simulink model "Disturbance"  (R2023b)
settings: Solver=VariableStepAuto  StartTime=0.0  StopTime=10.0  RelTol=1e-3
settings Model: Creator=hp  LastModifiedBy=hp

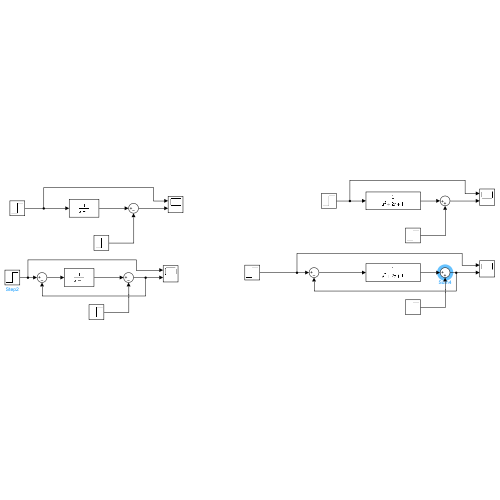
[thumbnail: Simulink's stored preview of the top-level diagram]
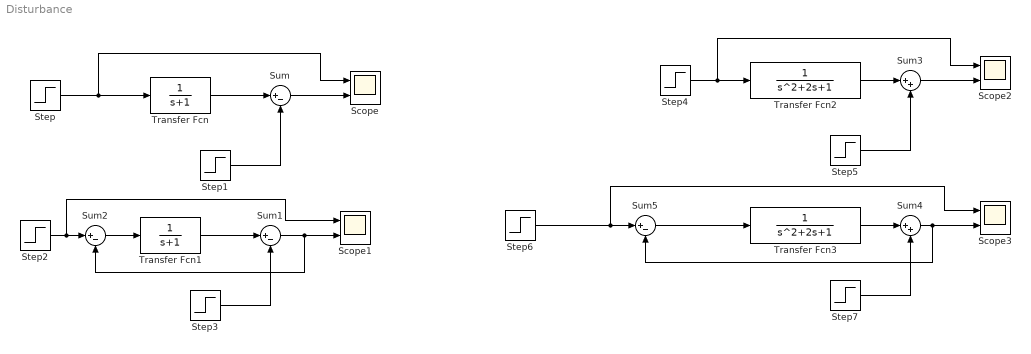
== system Disturbance ==
  Scope{,1..3} (4 alike) : Scope  NumInputPorts=2
  Step{,2,4,6} (4 alike) : Step  SampleTime=0
  Step1 : Step  Time=3  After=0.5  SampleTime=0
  Step3 : Step  Time=3  After=0.5  SampleTime=0
  Step5 : Step  Time=4  SampleTime=0.5
  Step7 : Step  Time=4  SampleTime=0.5
  Sum{,1..2,5} (4 alike) : Sum  Inputs=|+-
  Sum3 : Sum  Inputs=|++
  Sum4 : Sum  Inputs=|++
  Transfer Fcn : TransferFcn  Denominator=[1 1]
  Transfer Fcn1 : TransferFcn  Denominator=[1 1]
  Transfer Fcn2 : TransferFcn
  Transfer Fcn3 : TransferFcn
  wires:
  Transfer Fcn/1 -> Sum/1
  Sum/1 -> Scope/2
  Step1/1 -> Sum/2
  Step/1 -> Scope/1, Transfer Fcn/1
  Step3/1 -> Sum1/2
  Transfer Fcn1/1 -> Sum1/1
  Step2/1 -> Scope1/1, Sum2/1
  Sum2/1 -> Transfer Fcn1/1
  Sum1/1 -> Scope1/2, Sum2/2
  Step4/1 -> Scope2/1, Transfer Fcn2/1
  Transfer Fcn2/1 -> Sum3/1
  Step5/1 -> Sum3/2
  Sum3/1 -> Scope2/2
  Step7/1 -> Sum4/2
  Transfer Fcn3/1 -> Sum4/1
  Sum4/1 -> Scope3/2, Sum5/2
  Step6/1 -> Scope3/1, Sum5/1
  Sum5/1 -> Transfer Fcn3/1
